simulink model "ALGO_Corner_TrajTrack_MPC_T1_SP_LTR_Cosim_3D"  (R2023a)
settings: Solver=VariableStepAuto  StartTime=0.0  StopTime=12  RelTol=1e-3
values from neighbouring files (symbols this model uses):
  timeStep = 0.005    [Cosim_Setup_SLC_MPC_T1_SP_LTR_Cosim_3D.m]
libraries: simulink x7, Solver_SF x1
settings Model: Creator=QXJ  LastModifiedBy=28303
settings SolverCC: AlgebraicLoopSolver=TrustRegion
settings DebuggingCC: UnconnectedInputMsg=warning  UnconnectedOutputMsg=warning  UnconnectedLineMsg=warning
settings ModelReferenceCC: EnableRefExpFcnMdlSchedulingChecks=on
settings SFSimCC: CustomCodeUndefinedFunction=UseInterfaceOnly

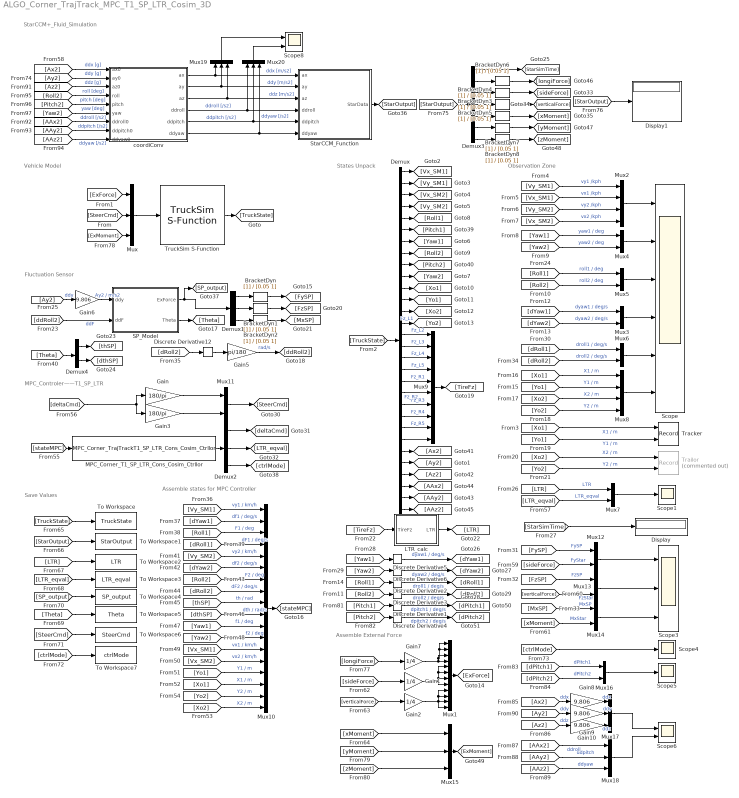
== system ALGO_Corner_TrajTrack_MPC_T1_SP_LTR_Cosim_3D ==
  note: Save Values
  note: StarCCM+_Fluid_Simulation
  note: MPC_Controler——T1_SP_LTR
  note: Assemble states for MPC Controller
  note: Observation Zone
  note: Vehicle Model
  note: Assemble External Force
  note: Fluctuation Sensor
  note: States Unpack
  BracketDyn{,1..8} (9 alike) : TransferFcn  Denominator=[0.05 1]
  Demux : Demux  Outputs=30
  Demux1 : Demux  Outputs=3
  Demux2 : Demux  Outputs=3
  Demux3 : Demux  Outputs=7
  Demux4 : Demux  Outputs=2
  Discrete Derivative{1..6,12} (7 alike) : simulink/Discrete/Discrete Derivative  gainval=1.0  ICPrevScaledInput=0.0  OutMin=[]  OutMax=[]  OutDataType=fixdt(1, 16)  OutScaling=2^-10  DoSatur=off
  Display : Display
  Display1 : Display
  Gain : Gain  Gain=180/pi
  Gain1 : Gain  Gain=1/4
  Gain{6,8..10} (4 alike) : Gain  Gain=9.806
  Gain2 : Gain  Gain=1/4
  Gain3 : Gain  Gain=180/pi
  Gain5 : Gain  Gain=pi/180
  Gain7 : Gain  Gain=1/4
  "LTR_calc " : MATLAB Function  TreatAsAtomicUnit=on
  MPC_Corner_T1_SP_LTR_Cons_Cosim_Ctrllor : S-Function  FunctionName=MPC_Corner_TrajTrackT1_SP_LTR_Cons_Cosim_Ctrllor  SFunctionDeploymentMode=off  EnableBusSupport=off
  Mux{,15,17..20} (6 alike) : Mux  Inputs=3
  Mux1 : Mux  Inputs=12
  Mux10 : Mux  Inputs=18
  Mux{3..7,11..14,16} (10 alike) : Mux  Inputs=2
  Mux2 : Mux
  Mux8 : Mux
  Mux9 : Mux  Inputs=10
  SP_Model : MATLAB Function  TreatAsAtomicUnit=on  SystemSampleTime=0.005
  Scope : Scope  NumInputPorts=6
  Scope1 : Scope
  Scope3 : Scope  NumInputPorts=3
  Scope4 : Scope
  Scope5 : Scope
  Scope6 : Scope  NumInputPorts=2
  Scope8 : Scope  NumInputPorts=2
  StarCCM_Function : MATLAB Function  TreatAsAtomicUnit=on  SystemSampleTime=[timeStep 0]
  To Workspace : ToWorkspace  VariableName=TruckState  SaveFormat=Timeseries  SampleTime=-1
  To Workspace1 : ToWorkspace  VariableName=StarOutput  SaveFormat=Timeseries  SampleTime=-1
  To Workspace2 : ToWorkspace  VariableName=LTR  SaveFormat=Timeseries  SampleTime=-1
  To Workspace3 : ToWorkspace  VariableName=LTR_eqval  SaveFormat=Timeseries  SampleTime=-1
  To Workspace4 : ToWorkspace  VariableName=SP_output  SaveFormat=Timeseries  SampleTime=-1
  To Workspace5 : ToWorkspace  VariableName=Theta  SaveFormat=Timeseries  SampleTime=-1
  To Workspace6 : ToWorkspace  VariableName=SteerCmd  SaveFormat=Timeseries  SampleTime=-1
  To Workspace7 : ToWorkspace  VariableName=ctrlMode  SaveFormat=Timeseries  SampleTime=-1
  Tracker : Record  FileSettingsInternal="{\"entries\":[{\"content\":{\"excelSettings\":{\"content\":{},\"type\":\"Streamout.ExcelSettings\"}},\"type\":\"Streamout.FileSettingStorage\",\"uuid\":\"7ae4536e-e7bc-4424-a4e1-f2e9e0387e01\"}],\"packageUris\":[\"http://schema.mathworks.com/mf0/streamout_blocks/R2020a\"],\"version\":\"1.0\"}"  Layout=[1 1]  SignalsInternal="{\"entries\":[{\"content\":{\"signals\":[{\"content\":{\"blockPath\":[\"ALGO_Corner_TrajTrack_MPC_T1_SP_LTR_Cosim_3D/Tracker\"],\"dimensions\":[1],\"domain\":\"ALGO_Corner_TrajTrack_MPC_T1_SP_LTR_Cosim_3D/Tracker\",\"lineColor\":\"#a2142f\",\"plots\":[1],\"port\":1,\"signalID\":16,\"signalName\":\"X1 / m\"},\"type\":\"RecordBlkView.Signal\",\"uuid\":\"78f39a7f-c97b-47b8-a87e-915073ed88bb\"},{\"content\":{\"blockPath\":[\"ALGO_Corner_TrajTrack_MPC_T1_SP_LTR_Cosim_3D/Tracker\"],\"dimensions\":[1],\"domain\":\"ALGO_Corner_TrajTrack_MPC_T1_SP_LTR_Cosim_3D/Tracker\",\"lineColor\":\"#139fff\",\"plots\":[1],\"port\":2,\"signalID\":19,\"signalName\":\"Y1 / m\"},\"type\":\"RecordBlkView.Signal\",\"uuid\":\"8d5dd065-9d53-452c-8f9c-36345176416b\"}]},\"type\":\"RecordBlkView.InputSignals\",\"uuid\":\"e477efe4-56bb-4c59-9738-f814d7dc8dcb\"}],\"packageUris\":[\"http://schema.mathworks.com/mf0/streamout_blocks/R2020a\"],\"version\":\"1.0\"}"  VisualizationBindings="{\"xyplotplugin\":{\"info\":[{\"series\":[{\"bindingParametersList\":[{\"parameter\":\"X-Axis\",\"signalID\":16,\"signalName\":\"X1 \\/ m\"},{\"parameter\":\"Y-Axis\",\"signalID\":19,\"signalName\":\"Y1 \\/ m\"}],\"seriesID\":24138}],\"subplotID\":1}]}}"  CompatibilityTag=XY  st=-1
  "Trailor " : Record  Commented=on  FileSettingsInternal="{\"entries\":[{\"content\":{\"excelSettings\":{\"content\":{},\"type\":\"Streamout.ExcelSettings\"}},\"type\":\"Streamout.FileSettingStorage\",\"uuid\":\"4c0e0dd3-d7e3-4a41-911e-3527c59e3239\"}],\"packageUris\":[\"http://schema.mathworks.com/mf0/streamout_blocks/R2020a\"],\"version\":\"1.0\"}"  Layout=[1 1]  SignalsInternal="{\"entries\":[{\"content\":{\"signals\":[{\"content\":{\"blockPath\":[\"ALGO_Corner_TrajTrack_MPC_T1_SP_LTR_Cosim_3D/Trailor \"],\"dimensions\":[1],\"domain\":\"ALGO_Corner_TrajTrack_MPC_T1_SP_LTR_Cosim_3D/Trailor \",\"lineColor\":\"#a2142f\",\"plots\":[1],\"port\":1,\"signalID\":8,\"signalName\":\"XY Graph:1\"},\"type\":\"RecordBlkView.Signal\",\"uuid\":\"950392ac-f098-49cf-ad9d-31ae19f60618\"},{\"content\":{\"blockPath\":[\"ALGO_Corner_TrajTrack_MPC_T1_SP_LTR_Cosim_3D/Trailor \"],\"dimensions\":[1],\"domain\":\"ALGO_Corner_TrajTrack_MPC_T1_SP_LTR_Cosim_3D/Trailor \",\"lineColor\":\"#139fff\",\"plots\":[1],\"port\":2,\"signalID\":11,\"signalName\":\"XY Graph:2\"},\"type\":\"RecordBlkView.Signal\",\"uuid\":\"bc26e29b-6a9b-47b1-823d-f8a75cf5a9ca\"}]},\"type\":\"RecordBlkView.InputSignals\",\"uuid\":\"22eeee0e-4f92-40ef-a089-236453f8b832\"}],\"packageUris\":[\"http://schema.mathworks.com/mf0/streamout_blocks/R2020a\"],\"version\":\"1.0\"}"  VisualizationBindings="{\"xyplotplugin\":{\"info\":[{\"series\":[{\"bindingParametersList\":[{\"parameter\":\"X-Axis\",\"signalID\":8,\"signalName\":\"XY Graph:1\"},{\"parameter\":\"Y-Axis\",\"signalID\":11,\"signalName\":\"XY Graph:2\"}],\"seriesID\":18457}],\"subplotID\":1}]}}"  CompatibilityTag=XY  st=-1
  TruckSim S-Function : Solver_SF/TruckSim S-Function  Priority=1  SIMFILE=ALGO_Corner_Tanker_TrajTrack_MPC_T1_SP_LTR_Cosim_3D.sim
      settings: SourceProductName=TruckSim S-Function
  coordiConv : MATLAB Function  TreatAsAtomicUnit=on
  wires:
  TruckSim S-Function/1 -> [TruckState]
  Mux/1 -> TruckSim S-Function/1
  Discrete Derivative12/1 -> Gain5/1
  Demux4/2 -> [dthSP]
  Demux4/1 -> [thSP]
  [Theta] -> Demux4/1
  Gain6/1 -> SP_Model/1(ddy)  "Ay2 / m/s2"
  Gain5/1 -> [ddRoll2]  "rad/s"
  Gain2/1 -> Mux1/9, Mux1/10, Mux1/12, Mux1/11
  [dRoll2] -> Discrete Derivative12/1
  BracketDyn/1 -> [FySP]
  BracketDyn1/1 -> [FzSP]
  BracketDyn2/1 -> [MxSP]
  SP_Model/1(ExForce) -> [SP_output], Demux1/1
  [Ay2] -> Gain6/1  "ddy"
  Demux1/1 -> BracketDyn/1
  Demux1/2 -> BracketDyn1/1
  Demux1/3 -> BracketDyn2/1
  SP_Model/2(Theta) -> [Theta]
  Mux1/1 -> [ExForce]
  [Yo1] -> Mux8/2  "Y1 / m"
  [Roll1] -> Mux5/1  "roll1 / deg"
  Mux3/1 -> Scope/4
  [Vx_SM1] -> Mux2/2  "vx1 /kph"
  [dRoll1] -> Mux6/1  "droll1 / deg/s"
  [Xo1] -> Tracker/1  "X1 / m"
  [Roll2] -> Mux5/2  "roll2 / deg"
  Mux8/1 -> Scope/6
  [Yo1] -> Tracker/2  "Y1 / m"
  Mux6/1 -> Scope/5
  Mux2/1 -> Scope/1
  [Yo2] -> "Trailor "/2  "Y2 / m"
  [dYaw2] -> Mux3/2  "dyaw2 / deg/s"
  [Yaw2] -> Mux4/2  "yaw2 / deg"
  [Vx_SM2] -> Mux2/4  "vx2 /kph"
  Mux5/1 -> Scope/3
  [Xo1] -> Mux8/1  "X1 / m"
  [Yaw1] -> Mux4/1  "yaw1 / deg"
  [Vy_SM2] -> Mux2/3  "vy2 /kph"
  [dYaw1] -> Mux3/1  "dyaw1 / deg/s"
  [Yo2] -> Mux8/4  "Y2 / m"
  Mux4/1 -> Scope/2
  [Xo2] -> Mux8/3  "X2 / m"
  [Xo2] -> "Trailor "/1  "X2 / m"
  [Vy_SM1] -> Mux2/1  "vy1 /kph"
  [dRoll2] -> Mux6/2  "droll2 / deg/s"
  Demux/2 -> [Vy_SM1]
  Demux/4 -> [Vy_SM2]
  Demux/1 -> [Vx_SM1]
  Demux/3 -> [Vx_SM2]
  [TruckState] -> Demux/1
  Mux9/1 -> [TireFz]
  [TireFz] -> "LTR_calc "/1(TireFz)
  "LTR_calc "/1(LTR) -> [LTR]
  [Yaw2] -> Discrete Derivative6/1
  Discrete Derivative5/1 -> [dYaw1]  "dyaw1 / deg/s"
  [Yaw1] -> Discrete Derivative5/1
  Discrete Derivative6/1 -> [dYaw2]  "dyaw2 / deg/s"
  [Roll1] -> Discrete Derivative2/1
  [Roll2] -> Discrete Derivative3/1
  Discrete Derivative2/1 -> [dRoll1]  "droll1 / deg/s"
  Discrete Derivative3/1 -> [dRoll2]  "droll2 / deg/s"
  [ExForce] -> Mux/1
  [SteerCmd] -> Mux/2
  [Vy_SM1] -> Mux10/1  "vy1 / km/h"
  [dYaw1] -> Mux10/2  "df1 / deg/s"
  [Roll1] -> Mux10/3  "F1 / deg"
  [dRoll1] -> Mux10/4  "dF1 / deg/s"
  [Vy_SM2] -> Mux10/5  "vy2 / km/h"
  [dYaw2] -> Mux10/6  "df2 / deg/s"
  [Roll2] -> Mux10/7  "F2 / deg"
  [dRoll2] -> Mux10/8  "dF2 / deg/s"
  [thSP] -> Mux10/9  "th / rad"
  [dthSP] -> Mux10/10  "dth / rad/s"
  [Yaw1] -> Mux10/11  "f1 / deg"
  [Yaw2] -> Mux10/12  "f2 / deg"
  [Vx_SM1] -> Mux10/13  "vx1 / km/h"
  [Vx_SM2] -> Mux10/14  "vx2 / km/h"
  [Xo2] -> Mux10/18  "X2 / m"
  [Yo2] -> Mux10/17  "Y2 / m"
  [Xo1] -> Mux10/16  "X1 / m"
  [Yo1] -> Mux10/15  "Y1 / m"
  Mux10/1 -> [stateMPC]
  [stateMPC] -> MPC_Corner_T1_SP_LTR_Cons_Cosim_Ctrllor/1
  MPC_Corner_T1_SP_LTR_Cons_Cosim_Ctrllor/1 -> Demux2/1
  Mux11/1 -> [SteerCmd]
  Demux2/1 -> [deltaCmd]
  Gain/1 -> Mux11/1
  Gain3/1 -> Mux11/2
  [deltaCmd] -> Gain3/1, Gain/1
  Demux2/2 -> [LTR_eqval]
  [LTR] -> Mux7/1  "LTR"
  [LTR_eqval] -> Mux7/2  "LTR_eqval"
  Mux7/1 -> Scope1/1
  Demux3/1 -> [StarSimTime]
  StarCCM_Function/1(StarData) -> [StarOutput]
  [StarSimTime] -> Display/1
  [sideForce] -> Gain1/1
  [verticalForce] -> Gain2/1
  [FySP] -> Mux12/1  "FySP"
  [sideForce] -> Mux12/2  "FyStar"
  [FzSP] -> Mux13/1  "FzSP"
  [verticalForce] -> Mux13/2  "FzStar"
  [xMoment] -> Mux14/2  "MxStar"
  [MxSP] -> Mux14/1  "MxSP"
  Mux12/1 -> Scope3/1
  Mux13/1 -> Scope3/2
  Mux14/1 -> Scope3/3
  [TruckState] -> To Workspace/1
  [StarOutput] -> To Workspace1/1
  [LTR] -> To Workspace2/1
  [LTR_eqval] -> To Workspace3/1
  [SP_output] -> To Workspace4/1
  [Theta] -> To Workspace5/1
  [SteerCmd] -> To Workspace6/1
  BracketDyn4/1 -> [sideForce]
  BracketDyn3/1 -> [verticalForce]
  BracketDyn5/1 -> [xMoment]
  [ddRoll2] -> SP_Model/2(ddF)  "ddF"
  Demux2/3 -> [ctrlMode]
  [ctrlMode] -> To Workspace7/1
  [ctrlMode] -> Scope4/1
  [StarOutput] -> Demux3/1
  [StarOutput] -> Display1/1
  Demux/24 -> Mux9/10
  Demux/23 -> Mux9/9  "Fz_R5"
  Demux/22 -> Mux9/8  "Fz_R4"
  Demux/21 -> Mux9/7  "Fz_R3"
  Demux/20 -> Mux9/6  "Fz_R2"
  Demux/19 -> Mux9/5  "Fz_R1"
  Demux/18 -> Mux9/4  "Fz_L5"
  Demux/10 -> [Yaw2]
  Demux/9 -> [Pitch2]
  Demux/8 -> [Roll2]
  Demux/7 -> [Yaw1]
  Demux/6 -> [Pitch1]
  Demux/5 -> [Roll1]
  Demux/11 -> [Xo1]
  Demux/12 -> [Yo1]
  Demux/13 -> [Xo2]
  Demux/14 -> [Yo2]  "Fz_L1"
  Demux/15 -> Mux9/1  "Fz_L2"
  Demux/16 -> Mux9/2  "Fz_L3"
  Demux/17 -> Mux9/3  "Fz_L4"
  Demux/25 -> [Ax2]
  Demux/26 -> [Ay2]
  Demux/27 -> [Az2]
  Demux/28 -> [AAx2]
  Demux/29 -> [AAy2]
  Demux/30 -> [AAz2]
  BracketDyn6/1 -> [longiForce]
  Demux3/2 -> BracketDyn6/1
  Demux3/3 -> BracketDyn4/1
  Demux3/4 -> BracketDyn3/1
  Demux3/5 -> BracketDyn5/1
  BracketDyn7/1 -> [yMoment]
  BracketDyn8/1 -> [zMoment]
  Demux3/6 -> BracketDyn7/1
  Demux3/7 -> BracketDyn8/1
  [longiForce] -> Gain7/1
  Gain7/1 -> Mux1/3, Mux1/1, Mux1/2, Mux1/4
  Gain1/1 -> Mux1/8, Mux1/6, Mux1/5, Mux1/7
  [ExMoment] -> Mux/3
  Mux15/1 -> [ExMoment]
  [Pitch1] -> Discrete Derivative1/1
  [Pitch2] -> Discrete Derivative4/1
  Discrete Derivative1/1 -> [dPitch1]  "dpitch1 / deg/s"
  Discrete Derivative4/1 -> [dPitch2]  "dpitch2 / deg/s"
  [dPitch1] -> Mux16/1  "dPitch1"
  [dPitch2] -> Mux16/2  "dPitch2"
  Mux16/1 -> Scope5/1
  [AAy2] -> Mux18/2  "ddpitch"
  [AAx2] -> Mux18/1  "ddroll"
  [AAz2] -> Mux18/3  "ddyaw"
  [Ay2] -> Gain9/1  "ddy"
  [Ax2] -> Gain8/1  "ddx"
  [Az2] -> Gain10/1  "ddz"
  Gain8/1 -> Mux17/1  "ddx"
  Gain9/1 -> Mux17/2  "ddy"
  Gain10/1 -> Mux17/3  "ddz"
  Mux17/1 -> Scope6/1
  Mux18/1 -> Scope6/2
  [Ax2] -> coordiConv/1(ax0)  "ddx [g]"
  [Ay2] -> coordiConv/2(ay0)  "ddy [g]"
  [Az2] -> coordiConv/3(az0)  "ddz [g]"
  [AAx2] -> coordiConv/7(ddroll0)  "ddroll [/s2]"
  [AAy2] -> coordiConv/8(ddpitch0)  "ddpitch [/s2]"
  [AAz2] -> coordiConv/9(ddyaw0)  "ddyaw [/s2]"
  [Roll2] -> coordiConv/4(roll)  "roll [deg]"
  [Pitch2] -> coordiConv/5(pitch)  "pitch [deg]"
  [Yaw2] -> coordiConv/6(yaw)  "yaw [deg]"
  coordiConv/1(ax) -> StarCCM_Function/1(ax), Mux19/1  "ddx [m/s2]"
  coordiConv/2(ay) -> StarCCM_Function/2(ay), Mux19/2  "ddy [m/s2]"
  coordiConv/3(az) -> StarCCM_Function/3(az), Mux19/3  "ddz [m/s2]"
  coordiConv/4(ddroll) -> Mux20/1, StarCCM_Function/4(ddroll)  "ddroll [/s2]"
  coordiConv/5(ddpitch) -> Mux20/2, StarCCM_Function/5(ddpitch)  "ddpitch [/s2]"
  coordiConv/6(ddyaw) -> StarCCM_Function/6(ddyaw), Mux20/3  "ddyaw [/s2]"
  Mux19/1 -> Scope8/1
  Mux20/1 -> Scope8/2
  [yMoment] -> Mux15/2
  [xMoment] -> Mux15/1
  [zMoment] -> Mux15/3

== matlab function ALGO_Corner_TrajTrack_MPC_T1_SP_LTR_Cosim_3D/SP_Model ==
  data: ddy input; ExForce output; ddF input; Theta output
function [ExForce,Theta] = SP_Model(ddy,ddF)
persistent sim_param Ts y0
%% 定义摆
if isempty(Ts)
%SP模型，共5个参数拟合
% 参数 m1 h0 hp lp coeff
x=[10890,1.5,0.13,0.97,0.13];
% 获取参数
sim_param=getParam_SP(x);
%初始状态量
y0=zeros(9,1);
%采样时间
Ts=0.005;
end

y=y0;

%% 求解微分方程
dy=zeros(9,1);
dy(1)=y(2);
dy(2)=ddy;
dy(3)=(dy(2)-y(3))/Ts;
dy(4)=y(5);
dy(5)=ddF;
dy(6)=(dy(5)-y(6))/Ts;
dy(7)=y(8);
dy(8)=calc_ddth_SP(y,sim_param);
dy(9)=(dy(8)-y(9))/Ts;
y=y0+dy*Ts;
%% 计算三向力输出
[Fy,Fz,Mx]=calc_Fp_SP(y,sim_param);
ExForce=[Fy,Fz,Mx];
%% 更新状态量
y0=y;
th=y(7);
dth=y(8);
Theta=[th,dth];
end

%% 根据变量获取参数
function sim_param=getParam_SP(x)
%根据变量生成传输参数
TotMass=14462;
m1=x(1);%参数1
m0=TotMass-m1;
h0=x(2);%参数2
hp=x(3);%参数3
lp=x(4);%参数4
g=9.806;
coeff=x(5);%参数5
sim_param=[m0,m1,h0,hp,lp,g,coeff];
end

%% 求解三向力输出
function [Fy,Fz,Mx] = calc_Fp_SP(state,param)
% sim_param=[m0,m1,h0,hp,lp,g,coeff];
m0=param(1);
m1=param(2);
h0=param(3);
hp=param(4);
lp=param(5);
g=param(6);
% co=param(7);

% y=state(1);
% dy=state(2);
ddy=state(3);
f=state(4);
df=state(5);
ddf=state(6);
th=state(7);
dth=state(8);
ddth=state(9);

%定义运算符简写
sf=sin(f);
cf=cos(f);
s2=sin(th+f);
c2=cos(th+f);
L=lp+hp;
%定义质量块的 位置矢量
exh=0.77; %额外增加的高度是罐底到车轴心的高度
R0=[-(exh+h0)*sf,(exh+h0)*cf];

R1=[-(exh+L)*sf+lp*s2
    (exh+L)*cf-lp*c2];

ddRp0=[ddy-h0*cf*ddf+df^2*h0*sf
-h0*sf*ddf-h0*cf*df^2+g];

ddRp1=[ddy+ddf*(-L*cf+lp*c2)+ddth*(lp*c2)+df^2*(L*sf-lp*s2)+dth^2*(-lp*s2)+df*dth*(-2*lp*s2)
ddf*(-L*sf+lp*s2)+ddth*(lp*s2)+df^2*(-L*cf+lp*c2)+dth^2*(lp*c2)+df*dth*(2*lp*c2)+g];

Fp=m0*ddRp0+m1*ddRp1;
Fy=Fp(1)*cf-(-Fp(2))*sf;
Fz=(-Fp(2))*cf+Fp(1)*sf;
Mx0=(m0*(R0(1)*-ddRp0(2)+R0(2)*ddRp0(1)));
Mx1=(m1*(R1(1)*-ddRp1(2)+R1(2)*ddRp1(1)));

Mx=Mx0+Mx1;

end
%% 求解ddth
function ddth = calc_ddth_SP(state,param)
% sim_param=[m0,m1,h0,hp,lp,g,coeff];
% m0=param(1);
% m1=param(2);
% h0=param(3);
hp=param(4);
lp=param(5);
g=param(6);
co=param(7);

% y=state(1);
% dy=state(2);
ddy=state(3);
f=state(4);
df=state(5);
ddf=state(6);
th=state(7);
dth=state(8);
% ddth=state(9);


%定义运算符简写
s1=sin(th);
c1=cos(th);
s2=sin(th+f);
c2=cos(th+f);
L=lp+hp;

ddth=-(ddy*lp*c2+ddf*(-lp*L*c1+lp^2)-df^2*lp*L*s1+g*lp*s2)/(lp^2);
ddth=ddth-co*dth;

end

== matlab function ALGO_Corner_TrajTrack_MPC_T1_SP_LTR_Cosim_3D/LTR_calc  ==
  data: TireFz input; LTR output
function LTR = fcn(TireFz)
% 分配物理量
FzL=sum(TireFz(1:5));
FzR=sum(TireFz(6:10));
% 进行计算
LTR=(FzL-FzR)/(FzL+FzR);
end

== matlab function ALGO_Corner_TrajTrack_MPC_T1_SP_LTR_Cosim_3D/StarCCM_Function ==
  data: ax input; StarData output; ay input; az input; ddroll input; ddpitch input; ddyaw input
function StarData = StarCCM_Fun(ax,ay,az,ddroll,ddpitch,ddyaw)
%定义标志位路径
java_flag = 'java_flag.csv';
matlab_flag = 'matlab_flag.csv';
%定义输出文件路径
java_output = 'java_output.csv';
matlab_output = 'matlab_output.csv';

%状态1：从StarCCM+的输出文件中提取数据

DataConv=getLastLineNum(java_output);
StarData=DataConv(1:7);

%状态2：Simulink利用获得的数据进行下一个仿真步

%状态3：Simulink输出数据文件，暂停自身的仿真
Matlab_Data=[ax,ay,az,ddroll,ddpitch,ddyaw];
writeData(Matlab_Data,matlab_output);

%状态4：置位matlab_flag标志位，允许StarCCM+采集数据
setFlag(matlab_flag);

%状态5：不断检测java_flag标志位，等待StarCCM+仿真结束
while(~getFlag(java_flag))
end
resetFlag(java_flag)
%进入下一个循环，回到状态1

end
%*************函数writeData*****************
%参数：data，数值向量
%参数：dir,目标输出文件地址
%将data转换为精度30的字符串写入目标文件
%*****************************************
function writeData(data,dir)
len=length(data);
buffer=sprintf('%0.10f',data(1));
if(len>=2)
    for i=2:len
    buffer=[buffer ',' sprintf('%0.10f',data(i))];
    end
    str=buffer;
else
    str='';
end

fileID = fopen(dir,'w');
fwrite(fileID,str,'char');
fclose(fileID);

end

%*************函数getLastLineNum*****************
%参数：dir,标志位文件的路径
%返回值：data,获得数据文件的最后一行并转换为数字数组
%*****************************************
function data=getLastLineNum(dir)
str=readLastLine(dir);
data=stringSplit(str,',');
end

%*************函数stringSplit*****************
%参数：str,待分割的字符串
%参数：notion,字符，用于指定分割的字符
%返回值：data,字符串数组，将字符串按照指定方式分割
%*****************************************
function data=stringSplit(str,notion)
len=length(str);
splitPlace=0;
for i=1:len
if(str(i)==notion)
splitPlace=[splitPlace i];

end
end
splitNum=length(splitPlace);
splitPlace=[splitPlace len+1];

data=zeros(1,splitNum);
for i=1:splitNum
data(i)=real(str2double(str((splitPlace(i)+1):(splitPlace(i+1)-1))));
end

end
%*************函数readLastLine*****************
%参数：dir,标志位文件的路径
%返回值：lastLine,字符串，最后一行的内容
%*****************************************
function lastLine=readLastLine(dir)
fileID = fopen(dir,'r');     %# Open the file as a binary
lastLine = '';                   %# Initialize to empty
offset = 1;                      %# Offset from the end of file
fseek(fileID,-offset,'eof');        %# Seek to the file end, minus the offset
newChar = fread(fileID,1,'char');  %# Read one character
while (newChar~=10) | (offset == 1)
  lastLine = [newChar lastLine];   %# Add the character to a string
  offset = offset+1;
  fseek(fileID,-offset,'eof');        %# Seek to the file end, minus the offset
  newChar = fread(fileID,1,'char');  %# Read one character
end
fclose(fileID);  %# Close the file
end
%*************函数getFlag*****************
%参数：dir,标志位文件的路径
%返回值：flag,获得标志位文件的内容，返回一个字节
%标志位,文件内容为'1'(49)则flag为1
%文件内容为'0'(48)则flag为0（其他非'1'内容则flag也为0）
%*****************************************
function flag=getFlag(dir)
fileID = fopen(dir,'r');%,'n','UTF-8'
    A = fread(fileID,1,'char');
    if(A==49)
    flag=1;
    else 
    flag=0;
    end
fclose(fileID);
end
%*************函数setFlag*****************
%参数：dir,标志位文件的路径
%返回值：无
%作用：重置标志位文件内容为'1'(49)
%*****************************************
function setFlag(dir)
fileID = fopen(dir,'w');
fwrite(fileID,'1','char');
fclose(fileID);
end
%*************函数resetFlag*****************
%参数：dir,标志位文件的路径
%返回值：无
%作用：重置标志位文件内容为'0'(48)
%*****************************************
function resetFlag(dir)
fileID = fopen(dir,'w');
fwrite(fileID,'0','char');
fclose(fileID);
end

== matlab function ALGO_Corner_TrajTrack_MPC_T1_SP_LTR_Cosim_3D/coordiConv ==
  data: ax0 input; ax output; ay0 input; az0 input; roll input; pitch input; yaw input; ddroll0 input; ddpitch0 input; ddyaw0 input; ay output; az output; ddroll output; ddpitch output; ddyaw output
function [ax,ay,az,ddroll,ddpitch,ddyaw]= coordiConv(ax0,ay0,az0,roll, pitch, yaw,ddroll0,ddpitch0,ddyaw0)%输入的旋转是角度degree
persistent g
if isempty(g)
    g = 9.806;
end

vec = Rotation3D([0;0;g], roll, pitch, yaw);


ax = -(vec(1) + ax0*g);
ay = -(vec(2) + ay0*g);
az = -(vec(3) + az0*g);

ddroll = -ddroll0;
ddpitch = -ddpitch0;
ddyaw = -ddyaw0;

end


function vec = Rotation3D(vec0, roll, pitch, yaw)
    % 将角度从度转换为弧度
    roll = deg2rad(roll);
    pitch = deg2rad(pitch);
    yaw = deg2rad(yaw);

    % 创建绕x轴旋转的旋转矩阵（Roll）
    Rx = [1, 0, 0;
          0, cos(roll), -sin(roll);
          0, sin(roll), cos(roll)];

    % 创建绕y轴旋转的旋转矩阵（Pitch）
    Ry = [cos(pitch), 0, sin(pitch);
          0, 1, 0;
          -sin(pitch), 0, cos(pitch)];

    % 创建绕z轴旋转的旋转矩阵（Yaw）
    Rz = [cos(yaw), -sin(yaw), 0;
          sin(yaw), cos(yaw), 0;
          0, 0, 1];

    % 综合旋转矩阵
    R = Rz * Ry * Rx;

    % 应用旋转矩阵到向量
    vec = R * vec0;
end
